simulink model "usefulBlocks"  (Simulink 7.3)
settings: Solver=ode45  StartTime=0.0  StopTime=10.0  RelTol=1e-3
settings Model: Creator=Wang  LastModifiedBy=Wang

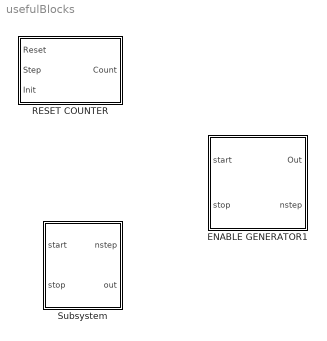
== system usefulBlocks ==
  ENABLE GENERATOR1 : Subsystem  RequirementInfo={} %GIDa_201a8ea9_ba15_4201_a60f_fd2c24b9582f  mask(CL_EnableGen){Out_type=High Active}
      mask prompts: Out_type "Pulse Type"
      mask help: Generate an enable signal between a start and a stop trigger. The output is normally off and it switches to on when the input start changes from 0 to 1. It remains on until the input end changes from 0 to 1, then switches again to off. If High Active is selected off =0, on = 1, viceversa for Low Active.
      mask init:
      | if (Out_type == 2), x = [0.65 0.65]; else x = [0.35,0.35]; end
      | if (Out_type == 2), y = [0.35 0.35]; else y = [0.65,0.65]; end
      | if (Out_type == 2), z = [0.35 0.35]; else z = [0.65,0.65]; end
      mask StyleString: popup(Low Active|High Active)
      mask Display:
      | plot([0.35 0.35],[0.65 0.35]);
      | plot([0.65 0.65],[0.65 0.35]);
      | 
      | plot([0.35 0.65],x);
      | plot([0.2 0.35],y);
      | plot([0.65 0.8],z);
      | 
      | plot([0.65 0.65],[0.23 0.31]);
      | plot([0.65 0.65],[0.11 0.19]);
      | plot([0.65 0.65],[0.69 0.77]);
      | plot([0.65 0.65],[0.81 0.89]);
      | plot([0.35 0.35],[0.23 0.31]);
      | plot([0.35 0.35],[0.11 0.19]);
      | plot([0.35 0.35],[0.69 0.77]);
      | plot([0.35 0.35],[0.81 0.89]);
      | 
      | plot([0 0.64], [0.21 0.21]);
      | plot([0.61 0.64], [0.18 0.21]);
      | plot([0.61 0.64], [0.24 0.21]);
      | 
      | plot([0 0.34], [0.78 0.78]);
      | plot([0.31 0.34], [0.75 0.78]);
      | plot([0.31 0.34], [0.8 0.78]);
      | 
      | text(0.04, 0.83, 'start','horizontalAlignment', 'left');
      | text(0.04, 0.3, 'end','horizontalAlignment', 'left');
      | text(0.99, 0.77, 'out','horizontalAlignment', 'right');
      | text(1, 0.25, 'nstep','horizontalAlignment', 'right');
  RESET COUNTER : Subsystem  RequirementInfo={} %GIDa_9b023074_786b_4ff2_be96_b9d3dceebbea
      mask Type: CL_ResetCount
      mask Description: Counter incremented with an input variable step (Step) and resettable with the input Reset to the input initial condition Init.
      mask Display:
      | plot([0.4 0.4 1],[0 0.3 0.3]);
      | text(0.45,0.22,'RESET');
      | text(0.45,0.08,'COUNTER');
  Subsystem : Subsystem

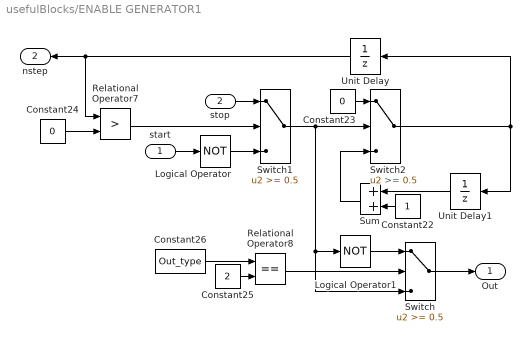
== system usefulBlocks/ENABLE GENERATOR1 ==
  start : Inport  RequirementInfo={} %GIDa_bf1e0d46_2d12_4316_bff8_9d4b8e7b89a2  OutDataType=sfix(16)  OutScaling=2^0
  stop : Inport  RequirementInfo={} %GIDa_4efaa4e2_974e_4a2a_a3c6_16de22efa608  Port=2  OutDataType=sfix(16)  OutScaling=2^0
  Constant22 : Constant  Tag=COPIED_DURING_UPGRADE  Description=|  RequirementInfo={} %GIDa_140a602d_ddda_4e51_8a82_6d76b95c8f87  OutDataType=sfix(16)  OutScaling=2^0  mask(TL_Constant){data={'date',734370.49190964119}}
      | Constant block of dSPACE TargetLink.
      | 
      | Output signal keeps the given constant value.
      settings: DeleteFcn=if exist('delete_tlblock','file')==2,delete_tlblock(gcbh);end  NameChangeFcn=if exist('rename_tlblock','file')==2,rename_tlblock(gcbh);end  OpenFcn=if exist('tl_open_blockdlg','file')==2,tl_open_blockdlg(gcbh);else,open_system(gcbh,'parameter');end
      mask Help: eval(['if exist(''tl_online_help'',''file'') == 2, tl_online_help(''Topic'',''TL_Constant''),else, web([''jar:file:///'',matlabroot,''/help/toolbox/simulink/help.jar!/slref/' lower(get_param(gcbh,'Blocktype')) '.html''], ''-helpbrowser''),end'])
      mask Display: plot([-0.05, 1.05, NaN, -0.05, 1.05],[.01, .01, NaN, .99, .99])
  Constant23 : Constant  Tag=COPIED_DURING_UPGRADE  Description=|  RequirementInfo={} %GIDa_130ccb9c_a41d_4794_abeb_d3dfa70ef9c2  Value=0  OutDataType=sfix(16)  OutScaling=2^0  mask(TL_Constant){data={'date',734370.49190927087}}
      | Constant block of dSPACE TargetLink.
      | 
      | Output signal keeps the given constant value.
      settings: DeleteFcn=if exist('delete_tlblock','file')==2,delete_tlblock(gcbh);end  NameChangeFcn=if exist('rename_tlblock','file')==2,rename_tlblock(gcbh);end  OpenFcn=if exist('tl_open_blockdlg','file')==2,tl_open_blockdlg(gcbh);else,open_system(gcbh,'parameter');end
      mask Help: eval(['if exist(''tl_online_help'',''file'') == 2, tl_online_help(''Topic'',''TL_Constant''),else, web([''jar:file:///'',matlabroot,''/help/toolbox/simulink/help.jar!/slref/' lower(get_param(gcbh,'Blocktype')) '.html''], ''-helpbrowser''),end'])
      mask Display: plot([-0.05, 1.05, NaN, -0.05, 1.05],[.01, .01, NaN, .99, .99])
  Constant24 : Constant  Tag=COPIED_DURING_UPGRADE  Description=|  RequirementInfo={} %GIDa_235a6bcb_563f_4ee2_a42c_c13b86915a99  Value=0  OutDataType=sfix(16)  OutScaling=2^0  mask(TL_Constant){data={'date',734370.49190891208}}
      | Constant block of dSPACE TargetLink.
      | 
      | Output signal keeps the given constant value.
      settings: DeleteFcn=if exist('delete_tlblock','file')==2,delete_tlblock(gcbh);end  NameChangeFcn=if exist('rename_tlblock','file')==2,rename_tlblock(gcbh);end  OpenFcn=if exist('tl_open_blockdlg','file')==2,tl_open_blockdlg(gcbh);else,open_system(gcbh,'parameter');end
      mask Help: eval(['if exist(''tl_online_help'',''file'') == 2, tl_online_help(''Topic'',''TL_Constant''),else, web([''jar:file:///'',matlabroot,''/help/toolbox/simulink/help.jar!/slref/' lower(get_param(gcbh,'Blocktype')) '.html''], ''-helpbrowser''),end'])
      mask Display: plot([-0.05, 1.05, NaN, -0.05, 1.05],[.01, .01, NaN, .99, .99])
  Constant25 : Constant  Tag=COPIED_DURING_UPGRADE  Description=|  RequirementInfo={} %GIDa_c2684536_7bed_4d43_aa10_4454bdcaa052  Value=2  OutDataType=sfix(16)  OutScaling=2^0  mask(TL_Constant){data={'date',734370.49190855329}}
      | Constant block of dSPACE TargetLink.
      | 
      | Output signal keeps the given constant value.
      settings: DeleteFcn=if exist('delete_tlblock','file')==2,delete_tlblock(gcbh);end  NameChangeFcn=if exist('rename_tlblock','file')==2,rename_tlblock(gcbh);end  OpenFcn=if exist('tl_open_blockdlg','file')==2,tl_open_blockdlg(gcbh);else,open_system(gcbh,'parameter');end
      mask Help: eval(['if exist(''tl_online_help'',''file'') == 2, tl_online_help(''Topic'',''TL_Constant''),else, web([''jar:file:///'',matlabroot,''/help/toolbox/simulink/help.jar!/slref/' lower(get_param(gcbh,'Blocktype')) '.html''], ''-helpbrowser''),end'])
      mask Display: plot([-0.05, 1.05, NaN, -0.05, 1.05],[.01, .01, NaN, .99, .99])
  Constant26 : Constant  Tag=COPIED_DURING_UPGRADE  Description=|  RequirementInfo={} %GIDa_46650ceb_5d6f_4809_b218_9cef489c7d16  Value=Out_type  OutDataType=sfix(16)  OutScaling=2^0  mask(TL_Constant){data={'date',734370.4919081945}}
      | Constant block of dSPACE TargetLink.
      | 
      | Output signal keeps the given constant value.
      settings: DeleteFcn=if exist('delete_tlblock','file')==2,delete_tlblock(gcbh);end  NameChangeFcn=if exist('rename_tlblock','file')==2,rename_tlblock(gcbh);end  OpenFcn=if exist('tl_open_blockdlg','file')==2,tl_open_blockdlg(gcbh);else,open_system(gcbh,'parameter');end
      mask Help: eval(['if exist(''tl_online_help'',''file'') == 2, tl_online_help(''Topic'',''TL_Constant''),else, web([''jar:file:///'',matlabroot,''/help/toolbox/simulink/help.jar!/slref/' lower(get_param(gcbh,'Blocktype')) '.html''], ''-helpbrowser''),end'])
      mask Display: plot([-0.05, 1.05, NaN, -0.05, 1.05],[.01, .01, NaN, .99, .99])
  Logical Operator : Logic  Tag=COPIED_DURING_UPGRADE  Description=|  RequirementInfo={} %GIDa_2cc13a48_13c8_4e59_adc7_b4052c8c31f2  Operator=NOT  Inputs=1  AllPortsSameDT=off  mask(TL_LogicalOperator){data={'logdata',{'plotchannels',[]},'date',734370.49190782406}}
      | Logical operator block of dSPACE TargetLink.
      | 
      | The Logical Operator block performs any of these logical operations on its inputs: AND, OR, NAND, NOR, XOR, and NOT. A nonzero input is treated as TRUE (1), a zero input as FALSE (0). The output depends on the selected operator. The output is 1 if TRUE and 0 if FALSE.
      settings: DeleteFcn=if exist('delete_tlblock','file')==2,delete_tlblock(gcbh);end  NameChangeFcn=if exist('rename_tlblock','file')==2,rename_tlblock(gcbh);end  OpenFcn=if exist('tl_open_blockdlg','file')==2,tl_open_blockdlg(gcbh);else,open_system(gcbh,'parameter');end
      mask Help: eval(['if exist(''tl_online_help'',''file'') == 2, tl_online_help(''Topic'',''TL_LogicalOperator''),else, web([''jar:file:///'',matlabroot,''/help/toolbox/simulink/help.jar!/slref/' lower(get_param(gcbh,'Blocktype')) '.html''], ''-helpbrowser''),end'])
      mask Display: plot([-0.05, 1.05, NaN, -0.05, 1.05],[.01, .01, NaN, .99, .99])
  Logical Operator1 : Logic  Tag=COPIED_DURING_UPGRADE  Description=|  RequirementInfo={} %GIDa_311ef1c0_6a13_4359_bd4e_03e82d6ad069  Operator=NOT  Inputs=1  AllPortsSameDT=off  mask(TL_LogicalOperator){data={'logdata',{'plotchannels',[]},'date',734370.49190765049}}
      | Logical operator block of dSPACE TargetLink.
      | 
      | The Logical Operator block performs any of these logical operations on its inputs: AND, OR, NAND, NOR, XOR, and NOT. A nonzero input is treated as TRUE (1), a zero input as FALSE (0). The output depends on the selected operator. The output is 1 if TRUE and 0 if FALSE.
      settings: DeleteFcn=if exist('delete_tlblock','file')==2,delete_tlblock(gcbh);end  NameChangeFcn=if exist('rename_tlblock','file')==2,rename_tlblock(gcbh);end  OpenFcn=if exist('tl_open_blockdlg','file')==2,tl_open_blockdlg(gcbh);else,open_system(gcbh,'parameter');end
      mask Help: eval(['if exist(''tl_online_help'',''file'') == 2, tl_online_help(''Topic'',''TL_LogicalOperator''),else, web([''jar:file:///'',matlabroot,''/help/toolbox/simulink/help.jar!/slref/' lower(get_param(gcbh,'Blocktype')) '.html''], ''-helpbrowser''),end'])
      mask Display: plot([-0.05, 1.05, NaN, -0.05, 1.05],[.01, .01, NaN, .99, .99])
  Relational Operator7 : RelationalOperator  Tag=COPIED_DURING_UPGRADE  Description=|  RequirementInfo={} %GIDa_98d1f3f6_e4e3_4bc2_9015_3baf934735f7  Operator=>  mask(TL_RelationalOperator){data={'logdata',{'plotchannels',[]},'date',734370.4919072917}}
      | Relational operator block of dSPACE TargetLink.
      | 
      | This block performs a relational operation on its two inputs u1 and u2 and produces output according to the following table.
      | If the result is TRUE, the output is 1; if FALSE, it is 0.
      | 
      | Operator   Output
      |  ==        TRUE if u1 is equal to u2
      |  !=        TRUE if u1 is not equal to u2
      |  <         TRUE if u1 is less than u2
      |  <=        TRUE if u1 is less than or equal to u2
      |  >=        TRUE if u1 is greater than or equal to u2
      |  >         TRUE if u1 is greater than u2
      settings: DeleteFcn=if exist('delete_tlblock','file')==2,delete_tlblock(gcbh);end  NameChangeFcn=if exist('rename_tlblock','file')==2,rename_tlblock(gcbh);end  OpenFcn=if exist('tl_open_blockdlg','file')==2,tl_open_blockdlg(gcbh);else,open_system(gcbh,'parameter');end
      mask Help: eval(['if exist(''tl_online_help'',''file'') == 2, tl_online_help(''Topic'',''TL_RelationalOperator''),else, web([''jar:file:///'',matlabroot,''/help/toolbox/simulink/help.jar!/slref/' lower(get_param(gcbh,'Blocktype')) '.html''], ''-helpbrowser''),end'])
      mask Display: plot([-0.05, 1.05, NaN, -0.05, 1.05],[.01, .01, NaN, .99, .99])
  Relational Operator8 : RelationalOperator  Tag=COPIED_DURING_UPGRADE  Description=|  RequirementInfo={} %GIDa_fb325a08_e4cc_42d3_b9a6_2acd92718822  Operator===  mask(TL_RelationalOperator){data={'logdata',{'plotchannels',[]},'date',734370.49190710648}}
      | Relational operator block of dSPACE TargetLink.
      | 
      | This block performs a relational operation on its two inputs u1 and u2 and produces output according to the following table.
      | If the result is TRUE, the output is 1; if FALSE, it is 0.
      | 
      | Operator   Output
      |  ==        TRUE if u1 is equal to u2
      |  !=        TRUE if u1 is not equal to u2
      |  <         TRUE if u1 is less than u2
      |  <=        TRUE if u1 is less than or equal to u2
      |  >=        TRUE if u1 is greater than or equal to u2
      |  >         TRUE if u1 is greater than u2
      settings: DeleteFcn=if exist('delete_tlblock','file')==2,delete_tlblock(gcbh);end  NameChangeFcn=if exist('rename_tlblock','file')==2,rename_tlblock(gcbh);end  OpenFcn=if exist('tl_open_blockdlg','file')==2,tl_open_blockdlg(gcbh);else,open_system(gcbh,'parameter');end
      mask Help: eval(['if exist(''tl_online_help'',''file'') == 2, tl_online_help(''Topic'',''TL_RelationalOperator''),else, web([''jar:file:///'',matlabroot,''/help/toolbox/simulink/help.jar!/slref/' lower(get_param(gcbh,'Blocktype')) '.html''], ''-helpbrowser''),end'])
      mask Display: plot([-0.05, 1.05, NaN, -0.05, 1.05],[.01, .01, NaN, .99, .99])
  Sum : Sum  Tag=COPIED_DURING_UPGRADE  Description=|  RequirementInfo={} %GIDa_fee237e1_540f_4031_b73c_44e11a4e403d  OutDataType=sfix(16)  OutScaling=2^-10  mask(TL_Sum){data={'logdata',{'plotchannels',[]},'output',{'type','UInt8'},'date',734370.49190674769}}
      | Sum block of dSPACE TargetLink.
      | 
      | Output signal is equal to the sum of the input signals.
      | The list of signs is specified according to conventions for Simulink Sum blocks.
      settings: DeleteFcn=if exist('delete_tlblock','file')==2,delete_tlblock(gcbh);end  NameChangeFcn=if exist('rename_tlblock','file')==2,rename_tlblock(gcbh);end  OpenFcn=if exist('tl_open_blockdlg','file')==2,tl_open_blockdlg(gcbh);else,open_system(gcbh,'parameter');end
      mask Help: eval(['if exist(''tl_online_help'',''file'') == 2, tl_online_help(''Topic'',''TL_Sum''),else, web([''jar:file:///'',matlabroot,''/help/toolbox/simulink/help.jar!/slref/' lower(get_param(gcbh,'Blocktype')) '.html''], ''-helpbrowser''),end'])
      mask Display: plot([-0.05, 1.05, NaN, -0.05, 1.05],[.01, .01, NaN, .99, .99])
  Switch : Switch  Tag=COPIED_DURING_UPGRADE  Description=|  RequirementInfo={} %GIDa_7150e51e_b68a_49bf_bdc2_b4a908e22df9  Threshold=0.5  OutDataType=sfix(16)  OutScaling=2^0  mask(TL_Switch){data={'logdata',{'plotchannels',[]},'output',{'max',1,'min',0,'type','UInt8'},'date',734370.49190637737}}
      | Switch block of dSPACE TargetLink.
      | 
      | Passes through input 1 if input 2 is greater than or equal to threshold, otherwise, passes through input 3:
      | 
      | if u2 >= threshold
      |    y = u1;
      | else
      |    y = u3;
      | end
      settings: DeleteFcn=if exist('delete_tlblock','file')==2,delete_tlblock(gcbh);end  NameChangeFcn=if exist('rename_tlblock','file')==2,rename_tlblock(gcbh);end  OpenFcn=if exist('tl_open_blockdlg','file')==2,tl_open_blockdlg(gcbh);else,open_system(gcbh,'parameter');end
      mask Help: eval(['if exist(''tl_online_help'',''file'') == 2, tl_online_help(''Topic'',''TL_Switch''),else, web([''jar:file:///'',matlabroot,''/help/toolbox/simulink/help.jar!/slref/' lower(get_param(gcbh,'Blocktype')) '.html''], ''-helpbrowser''),end'])
      mask Display: plot([-0.05, 1.05, NaN, -0.05, 1.05],[.01, .01, NaN, .99, .99])
  Switch1 : Switch  Tag=COPIED_DURING_UPGRADE  Description=|  RequirementInfo={} %GIDa_42f01913_5241_489c_9167_207469ef5ba8  Threshold=0.5  OutDataType=sfix(16)  OutScaling=2^0  mask(TL_Switch){data={'logdata',{'plotchannels',[]},'output',{'type','Bool'},'date',734370.49190584489}}
      | Switch block of dSPACE TargetLink.
      | 
      | Passes through input 1 if input 2 is greater than or equal to threshold, otherwise, passes through input 3:
      | 
      | if u2 >= threshold
      |    y = u1;
      | else
      |    y = u3;
      | end
      settings: DeleteFcn=if exist('delete_tlblock','file')==2,delete_tlblock(gcbh);end  NameChangeFcn=if exist('rename_tlblock','file')==2,rename_tlblock(gcbh);end  OpenFcn=if exist('tl_open_blockdlg','file')==2,tl_open_blockdlg(gcbh);else,open_system(gcbh,'parameter');end
      mask Help: eval(['if exist(''tl_online_help'',''file'') == 2, tl_online_help(''Topic'',''TL_Switch''),else, web([''jar:file:///'',matlabroot,''/help/toolbox/simulink/help.jar!/slref/' lower(get_param(gcbh,'Blocktype')) '.html''], ''-helpbrowser''),end'])
      mask Display: plot([-0.05, 1.05, NaN, -0.05, 1.05],[.01, .01, NaN, .99, .99])
  Switch2 : Switch  Tag=COPIED_DURING_UPGRADE  Description=|  RequirementInfo={} %GIDa_1bdd698b_9d07_4923_8591_3b150e34f272  Threshold=0.5  OutDataType=sfix(16)  OutScaling=2^0  mask(TL_Switch){data={'logdata',{'plotchannels',[]},'output',{'type','UInt8'},'date',734370.49190530088}}
      | Switch block of dSPACE TargetLink.
      | 
      | Passes through input 1 if input 2 is greater than or equal to threshold, otherwise, passes through input 3:
      | 
      | if u2 >= threshold
      |    y = u1;
      | else
      |    y = u3;
      | end
      settings: DeleteFcn=if exist('delete_tlblock','file')==2,delete_tlblock(gcbh);end  NameChangeFcn=if exist('rename_tlblock','file')==2,rename_tlblock(gcbh);end  OpenFcn=if exist('tl_open_blockdlg','file')==2,tl_open_blockdlg(gcbh);else,open_system(gcbh,'parameter');end
      mask Help: eval(['if exist(''tl_online_help'',''file'') == 2, tl_online_help(''Topic'',''TL_Switch''),else, web([''jar:file:///'',matlabroot,''/help/toolbox/simulink/help.jar!/slref/' lower(get_param(gcbh,'Blocktype')) '.html''], ''-helpbrowser''),end'])
      mask Display: plot([-0.05, 1.05, NaN, -0.05, 1.05],[.01, .01, NaN, .99, .99])
  Unit Delay : UnitDelay  Tag=COPIED_DURING_UPGRADE  Description=|  RequirementInfo={} %GIDa_fe8952cf_f4bd_47de_9ff7_3c67404d066a  SampleTime=-1  mask(TL_UnitDelay){data={'logdata',{'plotchannels',[]},'output',{'type','UInt8'},'state',{'type','UInt8'},'date',734370.49190475699}}
      | Unit Delay block of dSPACE TargetLink.
      | 
      | Output signal is equal to the input signal of the last sample step:
      | 
      |         y(k) = u(k-1).
      | 
      | In the 1st sampling step, the output signal is initialized with 'initial condition':
      | 
      |         y(0) = initial condition
      settings: DeleteFcn=if exist('delete_tlblock','file')==2,delete_tlblock(gcbh);end  NameChangeFcn=if exist('rename_tlblock','file')==2,rename_tlblock(gcbh);end  OpenFcn=if exist('tl_open_blockdlg','file')==2,tl_open_blockdlg(gcbh);else,open_system(gcbh,'parameter');end
      mask Help: eval(['if exist(''tl_online_help'',''file'') == 2, tl_online_help(''Topic'',''TL_UnitDelay''),else, web([''jar:file:///'',matlabroot,''/help/toolbox/simulink/help.jar!/slref/' lower(get_param(gcbh,'Blocktype')) '.html''], ''-helpbrowser''),end'])
      mask Display: plot([-0.05, 1.05, NaN, -0.05, 1.05],[.01, .01, NaN, .99, .99])
  Unit Delay1 : UnitDelay  Tag=COPIED_DURING_UPGRADE  Description=|  RequirementInfo={} %GIDa_896786c0_33c3_498d_9edc_2a3bf306746c  SampleTime=-1  mask(TL_UnitDelay){data={'logdata',{'plotchannels',[]},'output',{'type','UInt8'},'state',{'type','UInt8'},'date',734370.49190421298}}
      | Unit Delay block of dSPACE TargetLink.
      | 
      | Output signal is equal to the input signal of the last sample step:
      | 
      |         y(k) = u(k-1).
      | 
      | In the 1st sampling step, the output signal is initialized with 'initial condition':
      | 
      |         y(0) = initial condition
      settings: DeleteFcn=if exist('delete_tlblock','file')==2,delete_tlblock(gcbh);end  NameChangeFcn=if exist('rename_tlblock','file')==2,rename_tlblock(gcbh);end  OpenFcn=if exist('tl_open_blockdlg','file')==2,tl_open_blockdlg(gcbh);else,open_system(gcbh,'parameter');end
      mask Help: eval(['if exist(''tl_online_help'',''file'') == 2, tl_online_help(''Topic'',''TL_UnitDelay''),else, web([''jar:file:///'',matlabroot,''/help/toolbox/simulink/help.jar!/slref/' lower(get_param(gcbh,'Blocktype')) '.html''], ''-helpbrowser''),end'])
      mask Display: plot([-0.05, 1.05, NaN, -0.05, 1.05],[.01, .01, NaN, .99, .99])
  Out : Outport  RequirementInfo={} %GIDa_5eae2f49_d130_4534_8ff6_cbbdf149f5ce  OutDataType=sfix(16)  OutScaling=2^0
  nstep : Outport  RequirementInfo={} %GIDa_305dc0af_f935_4470_a1de_2d7fefb47190  Port=2  OutDataType=sfix(16)  OutScaling=2^0
  wires:
  Logical Operator/1 -> Switch1/3
  start/1 -> Logical Operator/1
  stop/1 -> Switch1/1
  Constant24/1 -> Relational Operator7/2
  Relational Operator7/1 -> Switch1/2
  Unit Delay/1 -> nstep/1, Relational Operator7/1
  Switch1/1 -> Logical Operator1/1, Switch/3, Switch2/2
  Constant25/1 -> Relational Operator8/2
  Constant26/1 -> Relational Operator8/1
  Relational Operator8/1 -> Switch/2
  Switch/1 -> Out/1
  Logical Operator1/1 -> Switch/1
  Sum/1 -> Switch2/3
  Constant23/1 -> Switch2/1
  Switch2/1 -> Unit Delay1/1, Unit Delay/1
  Constant22/1 -> Sum/2
  Unit Delay1/1 -> Sum/1

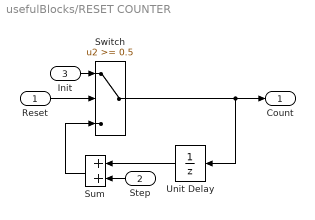
== system usefulBlocks/RESET COUNTER ==
  Reset : Inport  Tag=TYPE:; LSB:; OFF:; RANGE:; UNIT:;  RequirementInfo={} %GIDa_c61dec08_8ede_499e_a445_eb75b1d122e6  OutDataType=sfix(16)  OutScaling=2^0
  Step : Inport  Tag=TYPE:; LSB:; OFF:; RANGE:; UNIT:;  RequirementInfo={} %GIDa_dd6e2f10_a443_4764_816b_16ac24683437  Port=2  OutDataType=sfix(16)  OutScaling=2^0
  Init : Inport  Tag=TYPE:; LSB:; OFF:; RANGE:; UNIT:;  RequirementInfo={} %GIDa_08bdd9b5_c608_4eb1_8922_81aa6ce08049  Port=3  OutDataType=sfix(16)  OutScaling=2^0
  Sum : Sum  Tag=COPIED_DURING_UPGRADE  RequirementInfo={} %GIDa_a2e2d7e4_4922_48c8_a4be_fde9d9d04524  OutDataType=sfix(16)  OutScaling=2^0  SaturateOnIntegerOverflow=on  InputSameDT=on  OutDataTypeStr=Inherit: Same as first input  mask(TL_Sum){data={'logdata',{'plotchannels',[]},'output',{'type','UInt8'},'date',734370.49188685184}}
      settings: DeleteFcn=if exist('delete_tlblock','file')==2,delete_tlblock(gcbh);end  NameChangeFcn=if exist('rename_tlblock','file')==2,rename_tlblock(gcbh);end  OpenFcn=if exist('tl_open_blockdlg','file')==2,tl_open_blockdlg(gcbh);else,open_system(gcbh,'parameter');end
      mask Help: eval(['if exist(''tl_online_help'',''file'') == 2, tl_online_help(''Topic'',''TL_Sum''),else, web([''jar:file:///'',matlabroot,''/help/toolbox/simulink/help.jar!/slref/' lower(get_param(gcbh,'Blocktype')) '.html''], ''-helpbrowser''),end'])
      mask Display: plot([-0.05, 1.05, NaN, -0.05, 1.05],[.01, .01, NaN, .99, .99])
  Switch : Switch  Tag=COPIED_DURING_UPGRADE  RequirementInfo={} %GIDa_f80412b4_a0da_4926_af9f_3056622962d2  Threshold=0.5  OutDataType=sfix(16)  OutScaling=2^0  SaturateOnIntegerOverflow=on  InputSameDT=on  mask(TL_Switch){data={'logdata',{'plotchannels',[]},'output',{'type','UInt8'},'date',734370.49188630783}}
      settings: DeleteFcn=if exist('delete_tlblock','file')==2,delete_tlblock(gcbh);end  NameChangeFcn=if exist('rename_tlblock','file')==2,rename_tlblock(gcbh);end  OpenFcn=if exist('tl_open_blockdlg','file')==2,tl_open_blockdlg(gcbh);else,open_system(gcbh,'parameter');end
      mask Help: eval(['if exist(''tl_online_help'',''file'') == 2, tl_online_help(''Topic'',''TL_Switch''),else, web([''jar:file:///'',matlabroot,''/help/toolbox/simulink/help.jar!/slref/' lower(get_param(gcbh,'Blocktype')) '.html''], ''-helpbrowser''),end'])
      mask Display: plot([-0.05, 1.05, NaN, -0.05, 1.05],[.01, .01, NaN, .99, .99])
  Unit Delay : UnitDelay  Tag=COPIED_DURING_UPGRADE  RequirementInfo={} %GIDa_fad9a730_fae3_418f_9aff_087c033b2bd4  SampleTime=-1  mask(TL_UnitDelay){data={'logdata',{'plotchannels',[]},'output',{'type','UInt8'},'state',{'type','UInt8'},'date',734370.49188576394}}
      settings: DeleteFcn=if exist('delete_tlblock','file')==2,delete_tlblock(gcbh);end  NameChangeFcn=if exist('rename_tlblock','file')==2,rename_tlblock(gcbh);end  OpenFcn=if exist('tl_open_blockdlg','file')==2,tl_open_blockdlg(gcbh);else,open_system(gcbh,'parameter');end
      mask Help: eval(['if exist(''tl_online_help'',''file'') == 2, tl_online_help(''Topic'',''TL_UnitDelay''),else, web([''jar:file:///'',matlabroot,''/help/toolbox/simulink/help.jar!/slref/' lower(get_param(gcbh,'Blocktype')) '.html''], ''-helpbrowser''),end'])
      mask Display: plot([-0.05, 1.05, NaN, -0.05, 1.05],[.01, .01, NaN, .99, .99])
  Count : Outport  Tag=TYPE:; LSB:; OFF:; RANGE:; UNIT:;  RequirementInfo={} %GIDa_3665e323_aff5_41e1_ba42_81b3bd8e64b6  OutDataType=sfix(16)  OutScaling=2^0
  wires:
  Unit Delay/1 -> Sum/1
  Step/1 -> Sum/2
  Switch/1 -> Unit Delay/1, Count/1
  Reset/1 -> Switch/2
  Init/1 -> Switch/1
  Sum/1 -> Switch/3

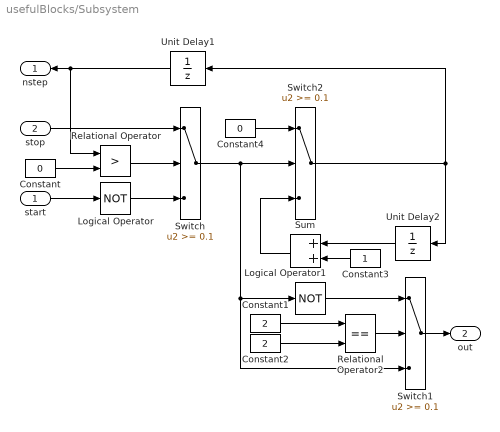
== system usefulBlocks/Subsystem ==
  start : Inport
  stop : Inport  Port=2
  Constant : Constant  Value=0  OutDataType=fixdt(1, 16)  OutScaling=2^0
  Constant1 : Constant  Value=2  OutDataType=fixdt(1, 16)  OutScaling=2^0
  Constant2 : Constant  Value=2  OutDataType=fixdt(1, 16)  OutScaling=2^0
  Constant3 : Constant  OutDataType=fixdt(1, 16)  OutScaling=2^0
  Constant4 : Constant  Value=0  OutDataType=fixdt(1, 16)  OutScaling=2^0
  Logical Operator : Logic  Operator=NOT  AllPortsSameDT=off  OutDataTypeMode=boolean  LogicDataType=fixdt(0, 8)  OutDataTypeStr=boolean
  Logical Operator1 : Logic  Operator=NOT  AllPortsSameDT=off  OutDataTypeMode=boolean  LogicDataType=fixdt(0, 8)  OutDataTypeStr=boolean
  Relational Operator : RelationalOperator  Operator=>  LogicOutDataTypeMode=boolean  LogicDataType=fixdt(0, 8)  OutDataTypeStr=boolean
  Relational Operator2 : RelationalOperator  Operator===  LogicOutDataTypeMode=boolean  LogicDataType=fixdt(0, 8)  OutDataTypeStr=boolean
  Sum : Sum  OutDataType=fixdt(1, 16)  OutScaling=2^0
  Switch : Switch  Threshold=0.1  OutDataType=fixdt(1, 16)  OutScaling=2^0  ZeroCross=off
  Switch1 : Switch  Threshold=0.1  OutDataType=fixdt(1, 16)  OutScaling=2^0
  Switch2 : Switch  Threshold=0.1  OutDataType=fixdt(1, 16)  OutScaling=2^0  ZeroCross=off
  Unit Delay1 : UnitDelay  SampleTime=-1
  Unit Delay2 : UnitDelay  X0=1  SampleTime=-1
  nstep : Outport
  out : Outport  Port=2
  wires:
  Logical Operator/1 -> Switch/3
  Relational Operator/1 -> Switch/2
  Unit Delay1/1 -> Relational Operator/1, nstep/1
  Constant/1 -> Relational Operator/2
  Unit Delay2/1 -> Sum/1
  Constant3/1 -> Sum/2
  Relational Operator2/1 -> Switch1/2
  Switch2/1 -> Unit Delay1/1, Unit Delay2/1
  Constant4/1 -> Switch2/1
  Switch/1 -> Switch2/2, Switch1/3, Logical Operator1/1
  Sum/1 -> Switch2/3
  Constant2/1 -> Relational Operator2/2
  Constant1/1 -> Relational Operator2/1
  Logical Operator1/1 -> Switch1/1
  stop/1 -> Switch/1
  start/1 -> Logical Operator/1
  Switch1/1 -> out/1
